simulink model "ACC2021_PositiveSystem_Delayed_Saturated"  (R2021a)
settings: Solver=ode1  StartTime=0.0  StopTime=60  FixedStep=1e-3  MaxStep=0.01  MinStep=0.001  RelTol=1e-3  AbsTol=1e-3
settings Model: Creator=s.ghetmiri  LastModifiedBy=guanyunliu
settings SolverCC: AlgebraicLoopSolver=LineSearch
settings DebuggingCC: SFMachineParentedDataDiag=warning  UnderSpecifiedDimensionMsg=warning

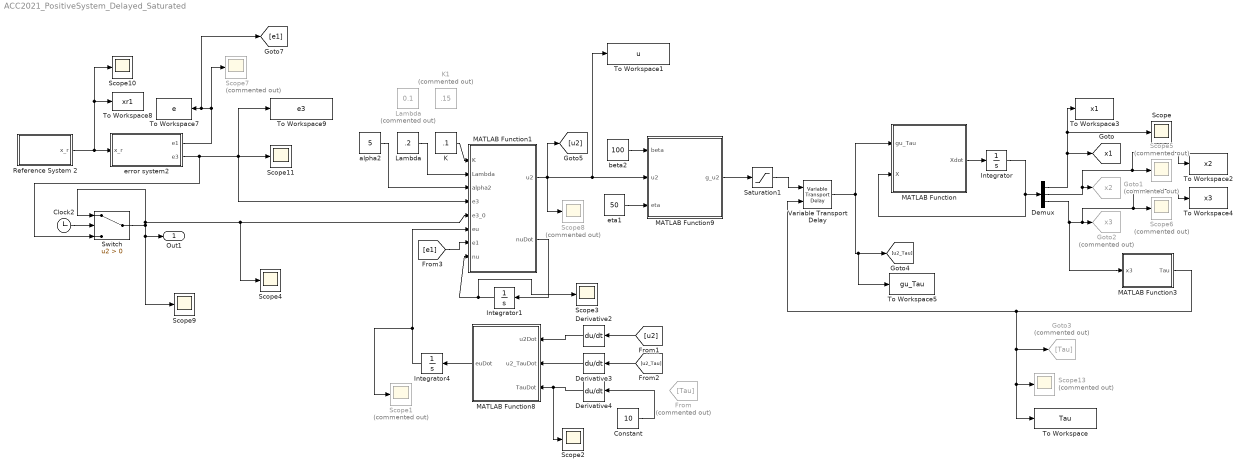
== system ACC2021_PositiveSystem_Delayed_Saturated ==
  Clock2 : Clock
  Constant : Constant  Value=10
  Demux : Demux  Outputs=3
  Derivative2 : Derivative  CoefficientInTFapproximation=0
  Derivative3 : Derivative  CoefficientInTFapproximation=0
  Derivative4 : Derivative  CoefficientInTFapproximation=0
  From : From  Commented=on  GotoTag=Tau
  Goto1 : Goto  Commented=on  GotoTag=x2  TagVisibility=global
  Goto2 : Goto  Commented=on  GotoTag=x3  TagVisibility=global
  Goto3 : Goto  Commented=on  GotoTag=Tau
  Integrator : Integrator  InitialCondition=[500;75;75]
  Integrator1 : Integrator
  Integrator4 : Integrator  InitialCondition=0.1
  K : Constant  Value=.1
  K1 : Constant  Commented=on  Value=.15
  Lambda : Constant  Commented=on  Value=0.1
  "Lambda " : Constant  Value=.2
  MATLAB Function : MATLAB Function  TreatAsAtomicUnit=on
  MATLAB Function1 : MATLAB Function  TreatAsAtomicUnit=on
  MATLAB Function3 : MATLAB Function  TreatAsAtomicUnit=on
  MATLAB Function8 : MATLAB Function  TreatAsAtomicUnit=on
  MATLAB Function9 : MATLAB Function  TreatAsAtomicUnit=on
  Reference System 2 : Subsystem
  Saturation1 : Saturate  UpperLimit=50  LowerLimit=0
  Scope{,2..4,9..11} (7 alike) : Scope
  Scope{1,5..8,13} (6 alike) : Scope  Commented=on
  Switch : Switch  Criteria=u2 > Threshold
  To Workspace : ToWorkspace  VariableName=Tau  SaveFormat=Timeseries  SampleTime=-1
  To Workspace1 : ToWorkspace  VariableName=u  SaveFormat=Timeseries  SampleTime=-1
  To Workspace2 : ToWorkspace  VariableName=x2  SaveFormat=Timeseries  SampleTime=-1
  To Workspace3 : ToWorkspace  VariableName=x1  SaveFormat=Timeseries  SampleTime=-1
  To Workspace4 : ToWorkspace  VariableName=x3  SaveFormat=Timeseries  SampleTime=-1
  To Workspace5 : ToWorkspace  VariableName=gu_Tau  SaveFormat=Timeseries  SampleTime=-1
  To Workspace7 : ToWorkspace  VariableName=e  SaveFormat=Timeseries  SampleTime=-1
  To Workspace8 : ToWorkspace  VariableName=xr1  SaveFormat=Timeseries  SampleTime=-1
  To Workspace9 : ToWorkspace  VariableName=e3  SaveFormat=Timeseries  SampleTime=-1
  Variable Transport Delay : VariableTransportDelay  VariableDelayType=Variable transport delay  MaximumDelay=10  MaximumPoints=10240
  alpha2 : Constant  Value=5
  "beta2 " : Constant  Value=100
  error system2 : Subsystem
  eta1 : Constant  Value=50
  Out1 : Outport
  tag scope: x1=global
  wires:
  MATLAB Function/1(Xdot) -> Integrator/1
  Integrator/1 -> MATLAB Function/2(X), Demux/1
  Demux/1 -> To Workspace3/1, Scope/1, [x1]
  Demux/2 -> To Workspace2/1, Scope5/1, Goto1/1
  MATLAB Function1/2(nuDot) -> Integrator1/1
  Integrator1/1 -> Scope3/1, MATLAB Function1/8(nu)
  alpha2/1 -> MATLAB Function1/3(alpha2)
  Derivative4/1 -> Scope2/1, MATLAB Function8/3(TauDot)
  [u2_Tau] -> Derivative3/1
  Derivative3/1 -> MATLAB Function8/2(u2_TauDot)
  [u2] -> Derivative2/1
  Derivative2/1 -> MATLAB Function8/1(u2Dot)
  MATLAB Function8/1(euDot) -> Integrator4/1
  MATLAB Function3/1(Tau) -> To Workspace/1, Scope13/1, Goto3/1, Variable Transport Delay/2
  Integrator4/1 -> Scope1/1, MATLAB Function1/6(eu)
  Reference System 2/1(x_r) -> To Workspace8/1, Scope10/1, error system2/1(x_r)
  error system2/1(e1) -> Scope7/1, [e1], To Workspace7/1
  error system2/2(e3) -> Switch/3, To Workspace9/1, Scope11/1, MATLAB Function1/4(e3)
  Switch/1 -> Scope4/1, MATLAB Function1/5(e3_0), Switch/1, Scope9/1, Out1/1
  Clock2/1 -> Switch/2
  MATLAB Function1/1(u2) -> Scope8/1, To Workspace1/1, MATLAB Function9/2(u2), [u2]
  eta1/1 -> MATLAB Function9/3(eta)
  "beta2 "/1 -> MATLAB Function9/1(beta)
  [e1] -> MATLAB Function1/7(e1)
  Demux/3 -> MATLAB Function3/1(x3), To Workspace4/1, Scope6/1, Goto2/1
  Constant/1 -> Derivative4/1
  MATLAB Function9/1(g_u2) -> Saturation1/1
  Saturation1/1 -> Variable Transport Delay/1
  Variable Transport Delay/1 -> To Workspace5/1, [u2_Tau], MATLAB Function/1(gu_Tau)
  "Lambda "/1 -> MATLAB Function1/2(Lambda)
  K/1 -> MATLAB Function1/1(K)

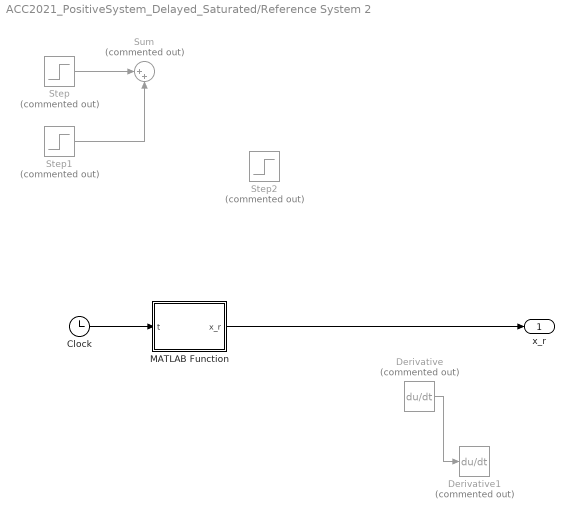
== system ACC2021_PositiveSystem_Delayed_Saturated/Reference System 2 ==
  Clock : Clock
  Derivative : Derivative  Commented=on
  Derivative1 : Derivative  Commented=on
  MATLAB Function : MATLAB Function  TreatAsAtomicUnit=on
  Step : Step  Commented=on  Time=2.4204  After=5  SampleTime=0
  Step1 : Step  Commented=on  Time=3.4204  After=-5  SampleTime=0
  Step2 : Step  Commented=on  After=3000  SampleTime=0
  Sum : Sum  Commented=on  Inputs=|++
  x_r : Outport
  wires:
  Step/1 -> Sum/1
  Step1/1 -> Sum/2
  Derivative/1 -> Derivative1/1
  Clock/1 -> MATLAB Function/1(t)
  MATLAB Function/1(x_r) -> x_r/1

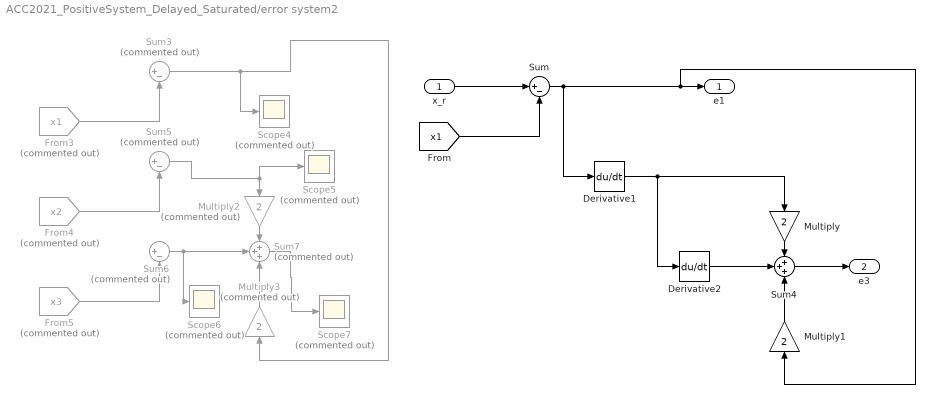
== system ACC2021_PositiveSystem_Delayed_Saturated/error system2 ==
  x_r : Inport
  Derivative1 : Derivative
  Derivative2 : Derivative
  From3 : From  Commented=on  GotoTag=x1  TagVisibility=global
  From4 : From  Commented=on  GotoTag=x2  TagVisibility=global
  From5 : From  Commented=on  GotoTag=x3  TagVisibility=global
  Multiply : Gain  Gain=2
  Multiply1 : Gain  Gain=2
  Multiply2 : Gain  Commented=on  Gain=2
  Multiply3 : Gain  Commented=on  Gain=2
  Scope{4..7} (4 alike) : Scope  Commented=on
  Sum : Sum  Inputs=|+-
  Sum3 : Sum  Commented=on  Inputs=|+-
  Sum4 : Sum  Inputs=+++
  Sum5 : Sum  Commented=on  Inputs=|+-
  Sum6 : Sum  Commented=on  Inputs=|+-
  Sum7 : Sum  Commented=on  Inputs=+++
  e1 : Outport
  e3 : Outport  Port=2
  wires:
  x_r/1 -> Sum/1
  [x1] -> Sum/2
  Sum/1 -> Derivative1/1, e1/1, Multiply1/1
  Derivative2/1 -> Sum4/2
  Multiply/1 -> Sum4/1
  Multiply1/1 -> Sum4/3
  Sum4/1 -> e3/1
  Multiply3/1 -> Sum7/3
  Multiply2/1 -> Sum7/1
  Sum6/1 -> Scope6/1, Sum7/2
  From5/1 -> Sum6/2
  From4/1 -> Sum5/2
  From3/1 -> Sum3/2
  Sum5/1 -> Scope5/1, Multiply2/1
  Sum7/1 -> Scope7/1
  Sum3/1 -> Scope4/1, Multiply3/1
  Derivative1/1 -> Derivative2/1, Multiply/1

== matlab function ACC2021_PositiveSystem_Delayed_Saturated/MATLAB Function1 ==
  data: K input; u2 output; Lambda input; alpha2 input; e3 input; e3_0 input; eu input; e1 input; nu input; nuDot output
function [u2, nuDot] = controller2(K,Lambda,alpha2,e3,e3_0,eu,e1,nu)

% u2=K*(e3-e3_0)+nu ;
% u2=K*(e3)+nu ;
% u2=abs(K*(e1)) ;

% u2=abs(K*(e3-e3_0)+nu) ;

if e1<=0
    u2=0;
else
    u2=K*(e3-e3_0)+nu ;
end

nuDot = K*(Lambda*e3+alpha2*eu) ;
return

== matlab function ACC2021_PositiveSystem_Delayed_Saturated/MATLAB Function ==
  data: Xdot output; gu_Tau input; X input
function Xdot = coagulation_model(gu_Tau, X)

a0=0.5370;
a1=2.4752;
a2=2.2306;
% b=154.1388;
b=1;

x1=X(1);
x2=X(2);
x3=X(3);


% x1dot=x2-a2*x1;
% x2dot=x3-a1*x1;
% x3dot=-a0*x1+b*(gu_Tau);

x1dot=x2-a2*x1;
x2dot=x3-.3*a1*x1;
x3dot=-.25*a0*x1+b*(gu_Tau);

Xdot=[x1dot;x2dot;x3dot];

== matlab function ACC2021_PositiveSystem_Delayed_Saturated/MATLAB Function3 ==
  data: x3 input; Tau output
function Tau = Delay(x3)


% Tau=(3*(max(x3,1)^(-0.25))) ;
% Tau=(0.0448*(max(x3,.202)^(-0.323))) ;
Tau=(4.48*(max(x3,.202)^(-0.323))) ;
% Tau=0;

== matlab function ACC2021_PositiveSystem_Delayed_Saturated/MATLAB Function8 ==
  data: u2Dot input; euDot output; u2_TauDot input; TauDot input
function euDot = eu_error(u2Dot,u2_TauDot, TauDot)

euDot = -u2Dot+(1-TauDot)*u2_TauDot;

== matlab function ACC2021_PositiveSystem_Delayed_Saturated/MATLAB Function9 ==
  data: beta input; u2 input; g_u2 output; eta input
function g_u2 = controller2_Sat(beta,u2,eta)

% g_u1 = (beta/2)+((beta/2)*tanh(Ks/2*(u1-eta)));
% Ks=8.4*(beta^-1.205);
% g_u2=1000+ 1000*tanh(8.8417e-4*(u1-2000))-56.572;
% g_u2 = ((beta/2)*tanh(Ks/2*(u2-eta)))-((beta/2)*tanh(Ks/2*(-eta)));
% g_u2 = (beta/2)+((beta/2)*tanh(Ks/2*(u2-eta)));
% g_u2 = ((beta/2+2)*tanh(Ks/2*(u2-eta)))-((beta/2)*tanh(Ks/2*(-eta)));
g_u2=u2; 
% g_u2 = (beta/2)+(beta/2)*tanh(Ks/2*(u2-eta));
Ks=0.022;
% g_u2 = (beta/2)+(beta/2)*tanh(Ks/2*(u2-eta));
return

== matlab function ACC2021_PositiveSystem_Delayed_Saturated/Reference System 2/MATLAB Function ==
  data: t input; x_r output
function x_r = fcn(t)

% x_r =(200*sin(.25*t)+300).*(1-exp(-t.^.5));

% x_r =(100*sin(.15*t)+300); 

x_r=200*(tanh(0.15*t)^2);
